simulink model "snac_openloop_SITL"  (R2024a)
settings: Solver=ode1  StartTime=0.0  StopTime=50  FixedStep=0.004  RelTol=1e-3  EnableMultiTasking=on
values from neighbouring files (symbols this model uses):
  x = bsxfun(@plus,x,settings.xoffset)    [NN7.m]
  y = bsxfun(@plus,y,settings.ymin)    [NN7.m]    (also in untitled2.m = r_smooth.r_smooth_1(1:3,:))
undefined symbols (not defined in the file or in its folder): DiscIntNeverNeededParam, vx, vy, vz, yaw, z
libraries: px4uORBlib x6, simulink x3, sharedtransform x1, px4lib x1
settings Model: ExtModeTrigDuration=10  Creator=re606359  LastModifiedBy=re606359
settings SolverCC: PositivePriorityOrder=on
settings OptimizationCC: EnhancedBackFolding=on  PassReuseOutputArgsAs=Individual arguments  ZeroExternalMemoryAtStartup=off  ZeroInternalMemoryAtStartup=off  MaxStackSize=64  OptimizeBlockOrder=speed  DifferentSizesBufferReuse=on  OptimizationCustomize=off  EfficientTunableParamExpr=on
settings DebuggingCC: ParameterTunabilityLossMsg=error
settings HardwareCC: ProdBitPerPointer=32  ProdBitPerSizeT=32  ProdBitPerPtrDiffT=32  ProdLargestAtomicInteger=Long  ProdLargestAtomicFloat=Double  ProdWordSize=32  ProdLongLongMode=on  ProdHWDeviceType=ARM Compatible->ARM Cortex
settings SFSimCC: MATLABDynamicMemAlloc=off  SimTargetLang=C++
settings RTWCC: Description=Embedded Coder  SystemTargetFile=ert.tlc  HardwareBoard=PX4 Host Target  TLCOptions="-aInlineSetEventsForThisBaseRateFcn=TLC_FALSE -aSuppressMultiTaskScheduler=TLC_FALSE  -aRateBasedStepFcn=0"  TemplateMakefile=ert_default_tmf  Toolchain=GNU Tools for PX4 Autopilots  PortableWordSizes=on  TargetLang=C++  GPUComputeCapability=3.5
settings CodeAppCC: ForceParamTrailComments=on  IgnoreCustomStorageClasses=off  OperatorAnnotations=on  SimulinkDataObjDesc=on  SFDataObjDesc=on  InsertBlockDesc=on
settings ERTTargetCC: SupportContinuousTime=on  ExtModeTransport=2  ExtModeStaticAlloc=on  ExtModeMexFile=ext_xcp  ExtModeIntrfLevel=Level2 - Open

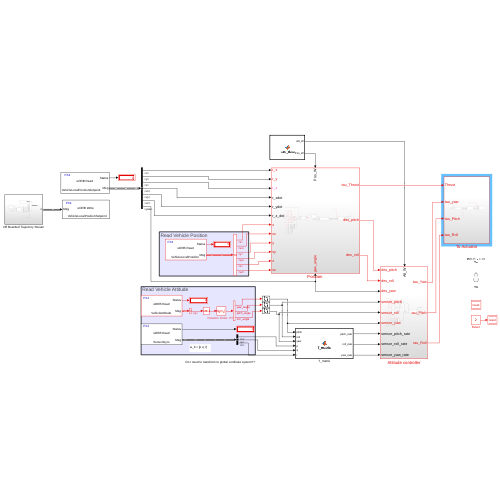
[thumbnail: Simulink's stored preview of the top-level diagram]
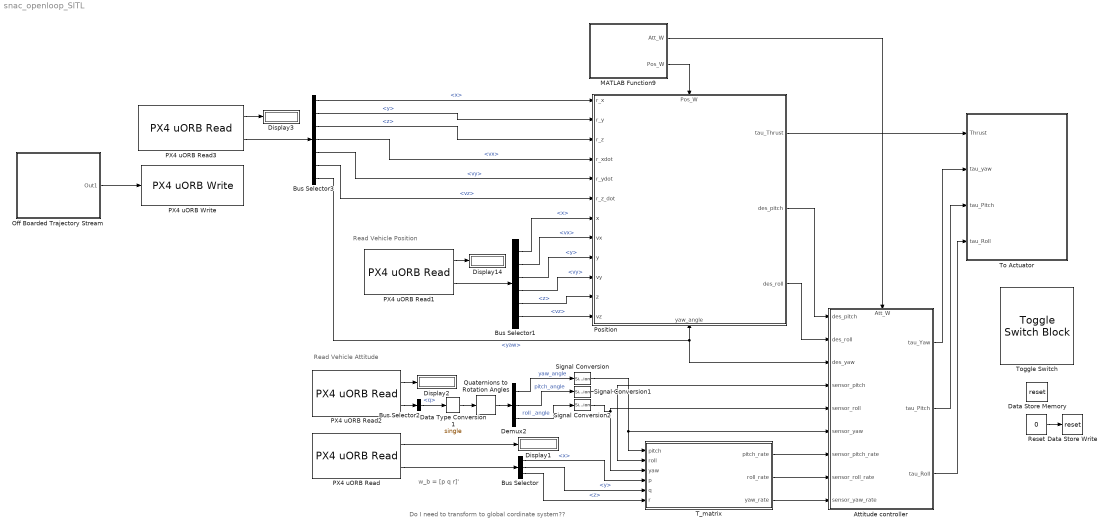
== system snac_openloop_SITL ==
  note: w_b = [p q r]'
  note: Read Vehicle Position
  note: Read Vehicle Attitude
  note: Do I need to transform to global cordinate system??
  Attitude controller : Subsystem
      settings: PortSchema="{\"entries\":[{\"content\":{\"sides\":[{\"content\":{\"connectorIds\":[\"In1\",\"In2\",\"In3\",\"In4\",\"In5\",\"In6\",\"In7\",\"In8\",\"In9\"]},\"type\":\"ConnectorPlacement.EquallySpacedRectSide\",\"uuid\":\"fae962e8-eaa0-4300-aebb-2542e8dc0b9d\"},{\"content\":{\"connectorIds\":[\"Out1\",\"Out2\",\"Out3\"],\"side\":\"RIGHT\"},\"type\":\"ConnectorPlacement.EquallySpacedRectSide\",\"uuid\":\"2ab64516-4178-4987-b105-e2b60ebc653b\"},{\"content\":{\"connectorIds\":[\"In10\"],\"side\":\"TOP\"},\"type\":\"ConnectorPlacement.EquallySpacedRectSide\",\"uuid\":\"8c218eee-bea7-4b7a-ab96-9bd58138bc2f\"},{\"content\":{\"side\":\"BOTTOM\"},\"type\":\"ConnectorPlacement.EquallySpacedRectSide\",\"uuid\":\"12c5faa8-5812-413f-bdcf-aa5ffbd59e54\"}]},\"type\":\"ConnectorPlacement.EquallySpacedConnector\",\"uuid\":\"49b20a1e-3c6c-4df6-a9b5-cb8878061c64\"}],\"packageUris\":[\"http://schema.mathworks.com/mf0/Connector/R2020b\"],\"version\":\"1.0\"}"
  Bus Selector : BusSelector  OutputSignals=x,y,z
  Bus Selector1 : BusSelector  OutputSignals=x,vx,y,vy,z,vz
  Bus Selector2 : BusSelector  OutputSignals=q
  Bus Selector3 : BusSelector  OutputSignals=x,y,z,vx,vy,vz,yaw
  Data Store Write : DataStoreWrite  DataStoreName=reset  IndexOptions=Index vector (dialog)  Indices=1  OutputSizes=1
  Data Store Memory : DataStoreMemory  DataStoreName=reset  ReadBeforeWriteMsg=warning  WriteAfterWriteMsg=warning  WriteAfterReadMsg=warning  ShowAdditionalParam=off  OutDataTypeStr=boolean
  Data Type Conversion1 : DataTypeConversion  OutDataTypeStr=single  SaturateOnIntegerOverflow=off  RndMeth=Floor
  Demux2 : Demux  Outputs=3
  Display{1..3,14} (4 alike) : Display
  MATLAB Function9 : MATLAB Function  TreatAsAtomicUnit=on
  Off Boarded Trajectory Stream : Subsystem
  PX4 uORB Read : px4uORBlib/PX4 uORB Read  uORBTopic=SensorGyro  selectInstance=SensorGyro  SampleTime=-1  BlockingMode=off  BlockTimeout=1e-3
  PX4 uORB Read1 : px4uORBlib/PX4 uORB Read  uORBTopic=VehicleLocalPosition  selectInstance=vehicle_local_position  SampleTime=-1  BlockingMode=off  BlockTimeout=1e-3
  PX4 uORB Read2 : px4uORBlib/PX4 uORB Read  uORBTopic=VehicleAttitude  selectInstance=vehicle_attitude  SampleTime=-1  BlockingMode=off  BlockTimeout=1e-3
  PX4 uORB Read3 : px4uORBlib/PX4 uORB Read  uORBTopic=VehicleLocalPositionSetpoint  selectInstance=VehicleLocalPositionSetpoint  SampleTime=-1  BlockingMode=off  BlockTimeout=1e-3
  PX4 uORB Write : px4uORBlib/PX4 uORB Write  uORBTopic=VehicleLocalPositionSetpoint  selectInstance=VehicleLocalPositionSetpoint  MessageQueueLen=1
  "Position " : Subsystem
      settings: PortSchema="{\"entries\":[{\"content\":{\"sides\":[{\"content\":{\"connectorIds\":[\"In1\",\"In2\",\"In3\",\"In4\",\"In5\",\"In6\",\"In7\",\"In8\",\"In9\",\"In10\",\"In11\",\"In12\"]},\"type\":\"ConnectorPlacement.EquallySpacedRectSide\",\"uuid\":\"96eb1e1d-33f8-43b2-aca1-3a2ea17c97d3\"},{\"content\":{\"connectorIds\":[\"Out1\",\"Out2\",\"Out3\"],\"side\":\"RIGHT\"},\"type\":\"ConnectorPlacement.EquallySpacedRectSide\",\"uuid\":\"68c63f59-0b7f-4dee-beff-edcde1fd911b\"},{\"content\":{\"connectorIds\":[\"In13\"],\"side\":\"TOP\"},\"type\":\"ConnectorPlacement.EquallySpacedRectSide\",\"uuid\":\"695c40b8-e625-4f49-aae8-ed972e1604cc\"},{\"content\":{\"connectorIds\":[\"In14\"],\"side\":\"BOTTOM\"},\"type\":\"ConnectorPlacement.EquallySpacedRectSide\",\"uuid\":\"eed3d45c-6018-4bc3-85c5-6c8aa0ab95cc\"}]},\"type\":\"ConnectorPlacement.EquallySpacedConnector\",\"uuid\":\"b4b28bb8-7674-4138-b24e-55baa1b4cc5c\"}],\"packageUris\":[\"http://schema.mathworks.com/mf0/Connector/R2020b\"],\"version\":\"1.0\"}"
  Quaternions to Rotation Angles : sharedtransform/Quaternions to Rotation Angles  rotationOrder=ZYX  aMode=aMode
  Reset : Constant  Value=0  OutDataTypeStr=boolean  SampleTime=-1
      settings: OpenFcn=|
      | if strcmp('0',get_param(gcb, 'Value'))                        set_param(gcb, 'Value', '1');
      | else
      |             set_param(gcb, 'Value', '0');
      | end
  Signal Conversion : SignalConversion  OverrideOpt=off
  Signal Conversion1 : SignalConversion  OverrideOpt=off
  Signal Conversion2 : SignalConversion  OverrideOpt=off
  T_matrix : MATLAB Function  TreatAsAtomicUnit=on
  To Actuator : Subsystem
  Toggle Switch : ToggleSwitchBlock
      settings: Values={{'Off', 'On'}, [0 1]}
  wires:
  Bus Selector1/3 -> "Position "/9(y)  "<y>"
  Demux2/3 -> Signal Conversion2/1  "roll _angle"
  Quaternions to Rotation Angles/1 -> Demux2/1
  PX4 uORB Read1/1 -> Display14/1
  Bus Selector3/6 -> "Position "/6(r_z_dot)  "<vz>"
  Bus Selector/3 -> T_matrix/6(r)  "<z>"
  Bus Selector1/6 -> "Position "/12(vz)  "<vz>"
  Bus Selector3/4 -> "Position "/4(r_xdot)  "<vx>"
  T_matrix/2(roll_rate) -> Attitude controller/8(sensor_roll_rate)
  T_matrix/1(pitch_rate) -> Attitude controller/7(sensor_pitch_rate)
  Demux2/2 -> Signal Conversion1/1  "pitch_angle"
  "Position "/3(des_roll) -> Attitude controller/2(des_roll)
  Bus Selector1/4 -> "Position "/10(vy)  "<vy>"
  Attitude controller/1(tau_Yaw) -> To Actuator/2(tau_yaw)
  Bus Selector3/2 -> "Position "/2(r_y)  "<y>"
  Bus Selector3/5 -> "Position "/5(r_ydot)  "<vy>"
  PX4 uORB Read2/1 -> Display2/1
  "Position "/1(tau_Thrust) -> To Actuator/1(Thrust)
  PX4 uORB Read2/2 -> Bus Selector2/1
  Bus Selector1/2 -> "Position "/8(vx)  "<vx>"
  PX4 uORB Read1/2 -> Bus Selector1/1
  Bus Selector/1 -> T_matrix/4(p)  "<x>"
  Data Type Conversion1/1 -> Quaternions to Rotation Angles/1
  MATLAB Function9/2(Pos_W) -> "Position "/13(Pos_W)
  PX4 uORB Read3/2 -> Bus Selector3/1
  Signal Conversion1/1 -> Attitude controller/4(sensor_pitch), T_matrix/2(roll)
  Bus Selector/2 -> T_matrix/5(q)  "<y>"
  Bus Selector3/3 -> "Position "/3(r_z)  "<z>"
  "Position "/2(des_pitch) -> Attitude controller/1(des_pitch)
  Bus Selector3/7 -> "Position "/14(yaw_angle), Attitude controller/3(des_yaw)  "<yaw>"
  Demux2/1 -> Signal Conversion/1  "yaw_angle"
  T_matrix/3(yaw_rate) -> Attitude controller/9(sensor_yaw_rate)
  Bus Selector1/1 -> "Position "/7(x)  "<x>"
  PX4 uORB Read/2 -> Bus Selector/1
  Attitude controller/2(tau_Pitch) -> To Actuator/3(tau_Pitch)
  Bus Selector3/1 -> "Position "/1(r_x)  "<x>"
  Reset/1 -> Data Store Write/1
  Bus Selector1/5 -> "Position "/11(z)  "<z>"
  Attitude controller/3(tau_Roll) -> To Actuator/4(tau_Roll)
  PX4 uORB Read/1 -> Display1/1
  Bus Selector2/1 -> Data Type Conversion1/1  "<q>"
  Signal Conversion2/1 -> T_matrix/3(yaw), Attitude controller/5("sensor_roll ")
  PX4 uORB Read3/1 -> Display3/1
  Signal Conversion/1 -> T_matrix/1(pitch), Attitude controller/6(sensor_yaw)
  MATLAB Function9/1(Att_W) -> Attitude controller/10(Att_W)
  Off Boarded Trajectory Stream/1(Out1) -> PX4 uORB Write/1

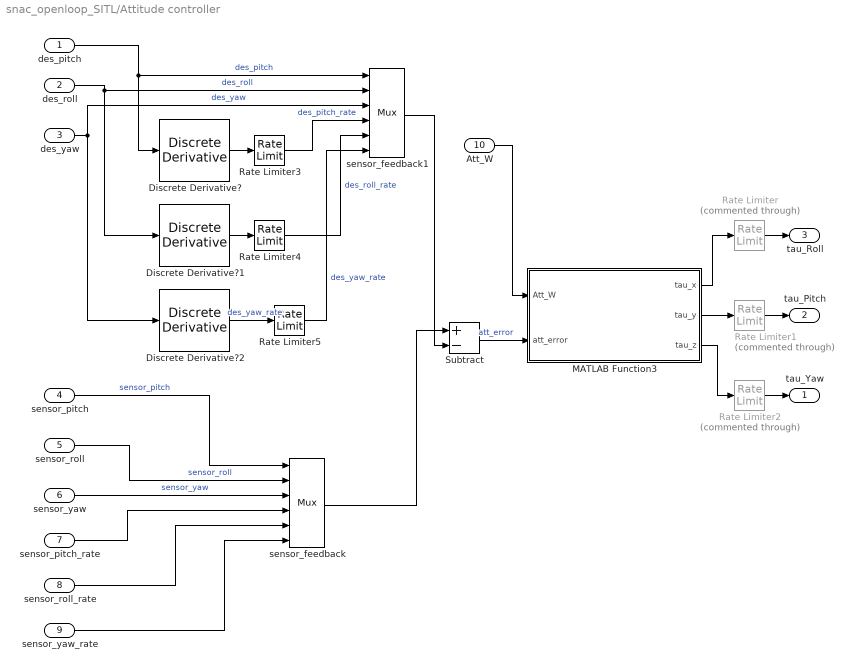
== system snac_openloop_SITL/Attitude controller ==
  des_pitch : Inport  OutDataTypeStr=single
  des_roll : Inport  Port=2  OutDataTypeStr=single
  des_yaw : Inport  Port=3  OutDataTypeStr=single
  sensor_pitch : Inport  Port=4
  "sensor_roll " : Inport  Port=5
  sensor_yaw : Inport  Port=6
  sensor_pitch_rate : Inport  Port=7
  sensor_roll_rate : Inport  Port=8
  sensor_yaw_rate : Inport  Port=9
  Att_W : Inport  Port=10
  Discrete Derivative? : simulink/Discrete/Discrete Derivative  gainval=1.0  ICPrevScaledInput=0.0  OutMin=[-5]  OutMax=[5]  OutDataTypeStr=single  OutputDataTypeScalingMode=single  OutDataType=fixdt(1, 16)  OutScaling=2^-10  DoSatur=off
  Discrete Derivative?1 : simulink/Discrete/Discrete Derivative  gainval=1.0  ICPrevScaledInput=0.0  OutMin=[-5]  OutMax=[5]  OutDataTypeStr=single  OutputDataTypeScalingMode=single  OutDataType=fixdt(1, 16)  OutScaling=2^-10  DoSatur=off
  Discrete Derivative?2 : simulink/Discrete/Discrete Derivative  gainval=1.0  ICPrevScaledInput=0.0  OutMin=[-2]  OutMax=[2]  OutDataTypeStr=single  OutputDataTypeScalingMode=single  OutDataType=fixdt(1, 16)  OutScaling=2^-10  DoSatur=off
  MATLAB Function3 : MATLAB Function  TreatAsAtomicUnit=on
  Rate Limiter : RateLimiter  Commented=through  RisingSlewLimit=2  FallingSlewLimit=-2  SampleTimeMode=inherited
  Rate Limiter1 : RateLimiter  Commented=through  RisingSlewLimit=2  FallingSlewLimit=-2  SampleTimeMode=inherited
  Rate Limiter2 : RateLimiter  Commented=through  RisingSlewLimit=2  FallingSlewLimit=-2  SampleTimeMode=inherited
  Rate Limiter3 : RateLimiter  RisingSlewLimit=2  FallingSlewLimit=-2  SampleTimeMode=inherited
  Rate Limiter4 : RateLimiter  RisingSlewLimit=2  FallingSlewLimit=-2  SampleTimeMode=inherited
  Rate Limiter5 : RateLimiter  RisingSlewLimit=2  FallingSlewLimit=-2  SampleTimeMode=inherited
  Subtract : Sum  Inputs=+-
  sensor_feedback : Mux  Inputs=6
  sensor_feedback1 : Mux  Inputs=6
  tau_Yaw : Outport
  tau_Pitch : Outport  Port=2
  tau_Roll : Outport  Port=3
  wires:
  sensor_pitch/1 -> sensor_feedback/1  "sensor_pitch"
  "sensor_roll "/1 -> sensor_feedback/2  "sensor_roll"
  sensor_yaw/1 -> sensor_feedback/3  "sensor_yaw"
  sensor_pitch_rate/1 -> sensor_feedback/4
  sensor_roll_rate/1 -> sensor_feedback/5
  sensor_yaw_rate/1 -> sensor_feedback/6
  Att_W/1 -> MATLAB Function3/1(Att_W)
  Subtract/1 -> MATLAB Function3/2(att_error)  "att_error"
  des_pitch/1 -> Discrete Derivative?/1, sensor_feedback1/1  "des_pitch"
  des_roll/1 -> Discrete Derivative?1/1, sensor_feedback1/2  "des_roll"
  des_yaw/1 -> Discrete Derivative?2/1, sensor_feedback1/3  "des_yaw"
  Rate Limiter5/1 -> sensor_feedback1/6  "des_yaw_rate"
  Rate Limiter4/1 -> sensor_feedback1/5  "des_roll_rate"
  Rate Limiter3/1 -> sensor_feedback1/4  "des_pitch_rate"
  sensor_feedback/1 -> Subtract/1
  sensor_feedback1/1 -> Subtract/2
  Discrete Derivative?1/1 -> Rate Limiter4/1
  Discrete Derivative?/1 -> Rate Limiter3/1
  Discrete Derivative?2/1 -> Rate Limiter5/1  "des_yaw_rate"
  MATLAB Function3/1(tau_x) -> Rate Limiter/1
  MATLAB Function3/2(tau_y) -> Rate Limiter1/1
  MATLAB Function3/3(tau_z) -> Rate Limiter2/1
  Rate Limiter/1 -> tau_Roll/1
  Rate Limiter1/1 -> tau_Pitch/1
  Rate Limiter2/1 -> tau_Yaw/1

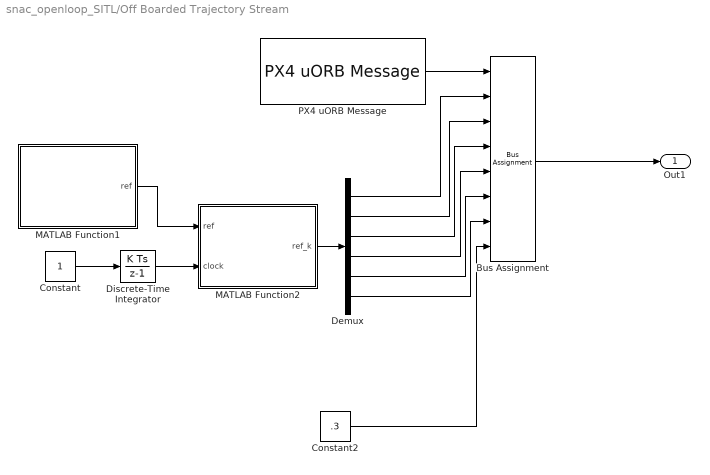
== system snac_openloop_SITL/Off Boarded Trajectory Stream ==
  Bus Assignment : BusAssignment  AssignedSignals=x,y,z,vx,vy,vz,yaw
  Constant : Constant  OutDataTypeStr=single
  Constant2 : Constant  Value=.3  OutDataTypeStr=single
  Demux : Demux  Outputs=6
  Discrete-Time Integrator : DiscreteIntegrator  SampleTime=-1  ICPrevOutput=DiscIntNeverNeededParam  ICPrevScaledInput=DiscIntNeverNeededParam
  MATLAB Function1 : MATLAB Function  TreatAsAtomicUnit=on
  MATLAB Function2 : MATLAB Function  TreatAsAtomicUnit=on
  PX4 uORB Message : px4uORBlib/PX4 uORB Message  uORBTopic=VehicleLocalPositionSetpoint  SampleTime=-1  selectInstance=VehicleLocalPositionSetpoint
  Out1 : Outport
  wires:
  MATLAB Function1/1(ref) -> MATLAB Function2/1(ref)
  Discrete-Time Integrator/1 -> MATLAB Function2/2(clock)
  Demux/2 -> Bus Assignment/3
  Demux/3 -> Bus Assignment/4
  PX4 uORB Message/1 -> Bus Assignment/1
  Demux/1 -> Bus Assignment/2
  Constant/1 -> Discrete-Time Integrator/1
  Demux/4 -> Bus Assignment/5
  Constant2/1 -> Bus Assignment/8
  Demux/5 -> Bus Assignment/6
  Demux/6 -> Bus Assignment/7
  MATLAB Function2/1(ref_k) -> Demux/1
  Bus Assignment/1 -> Out1/1

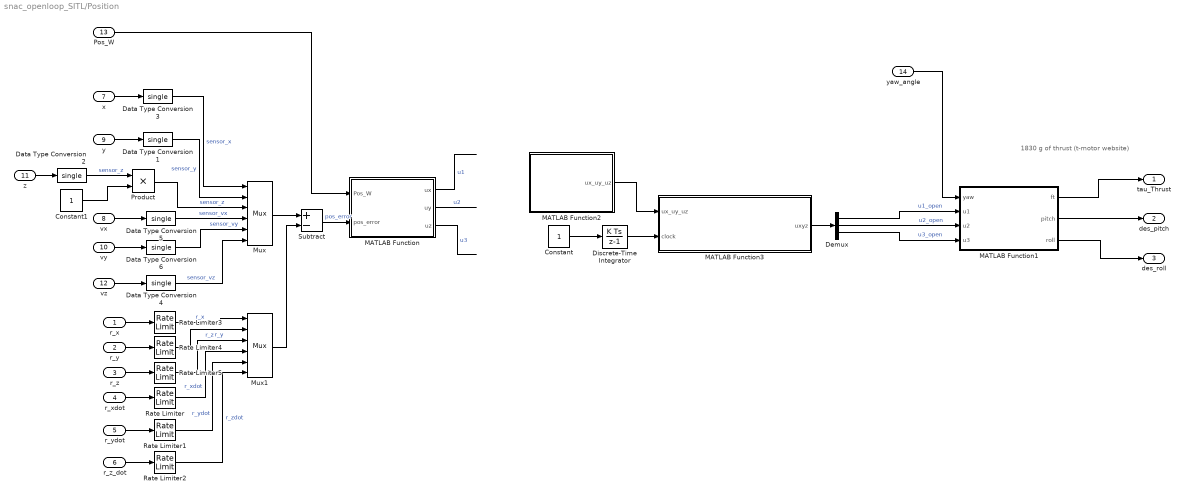
== system snac_openloop_SITL/Position  ==
  note: 1830 g of thrust (t-motor website)
  r_x : Inport
  r_y : Inport  Port=2
  r_z : Inport  Port=3
  r_xdot : Inport  Port=4
  r_ydot : Inport  Port=5
  r_z_dot : Inport  Port=6
  x : Inport  Port=7
  vx : Inport  Port=8
  y : Inport  Port=9
  vy : Inport  Port=10
  z : Inport  Port=11
  vz : Inport  Port=12
  Pos_W : Inport  Port=13
  yaw_angle : Inport  Port=14
  Constant : Constant  OutDataTypeStr=single
  Constant1 : Constant  OutDataTypeStr=single
  Data Type Conversion{1..6} (6 alike) : DataTypeConversion  OutDataTypeStr=single  SaturateOnIntegerOverflow=off  RndMeth=Floor
  Demux : Demux  Outputs=3
  Discrete-Time Integrator : DiscreteIntegrator  SampleTime=-1  ICPrevOutput=DiscIntNeverNeededParam  ICPrevScaledInput=DiscIntNeverNeededParam
  MATLAB Function : MATLAB Function  TreatAsAtomicUnit=on
  MATLAB Function1 : MATLAB Function  TreatAsAtomicUnit=on
  MATLAB Function2 : MATLAB Function  TreatAsAtomicUnit=on
  MATLAB Function3 : MATLAB Function  TreatAsAtomicUnit=on
  Mux : Mux  Inputs=6
  Mux1 : Mux  Inputs=6
  Product : Product
  Rate Limiter{,1..5} (6 alike) : RateLimiter  RisingSlewLimit=15  FallingSlewLimit=-15  SampleTimeMode=inherited
  Subtract : Sum  Inputs=+-
  tau_Thrust : Outport  OutDataTypeStr=single
  des_pitch : Outport  Port=2
  des_roll : Outport  Port=3
  wires:
  z/1 -> Data Type Conversion2/1
  x/1 -> Data Type Conversion3/1
  y/1 -> Data Type Conversion1/1
  vz/1 -> Data Type Conversion4/1
  vx/1 -> Data Type Conversion5/1
  vy/1 -> Data Type Conversion6/1
  Pos_W/1 -> MATLAB Function/1(Pos_W)
  Data Type Conversion3/1 -> Mux/1  "sensor_x"
  Data Type Conversion1/1 -> Mux/2  "sensor_y"
  Data Type Conversion5/1 -> Mux/4  "sensor_vx"
  Data Type Conversion6/1 -> Mux/5  "sensor_vy"
  Data Type Conversion4/1 -> Mux/6  "sensor_vz"
  Mux/1 -> Subtract/1
  Mux1/1 -> Subtract/2
  Subtract/1 -> MATLAB Function/2(pos_error)  "pos_error"
  Demux/1 -> MATLAB Function1/2(u1)  "u1_open"
  Demux/2 -> MATLAB Function1/3(u2)  "u2_open"
  Demux/3 -> MATLAB Function1/4(u3)  "u3_open"
  yaw_angle/1 -> MATLAB Function1/1(yaw)
  r_ydot/1 -> Rate Limiter1/1
  r_z_dot/1 -> Rate Limiter2/1
  r_xdot/1 -> Rate Limiter/1
  Rate Limiter/1 -> Mux1/4  "r_xdot"
  Rate Limiter1/1 -> Mux1/5  "r_ydot"
  Rate Limiter2/1 -> Mux1/6  "r_zdot"
  Data Type Conversion2/1 -> Product/1  "sensor_z"
  Product/1 -> Mux/3  "sensor_z"
  Constant1/1 -> Product/2
  r_x/1 -> Rate Limiter3/1
  Rate Limiter3/1 -> Mux1/1  "r_x"
  r_y/1 -> Rate Limiter4/1
  Rate Limiter4/1 -> Mux1/2  "r_y"
  r_z/1 -> Rate Limiter5/1
  Rate Limiter5/1 -> Mux1/3  "r_z"
  MATLAB Function1/1(ft) -> tau_Thrust/1
  MATLAB Function1/2(pitch) -> des_pitch/1
  MATLAB Function1/3(roll) -> des_roll/1
  MATLAB Function2/1(ux_uy_uz) -> MATLAB Function3/1(ux_uy_uz)
  Discrete-Time Integrator/1 -> MATLAB Function3/2(clock)
  Constant/1 -> Discrete-Time Integrator/1
  MATLAB Function3/1(uxyz) -> Demux/1
  MATLAB Function/3(uz) -> ?  "u3"
  MATLAB Function/1(ux) -> ?  "u1"
  MATLAB Function/2(uy) -> ?  "u2"

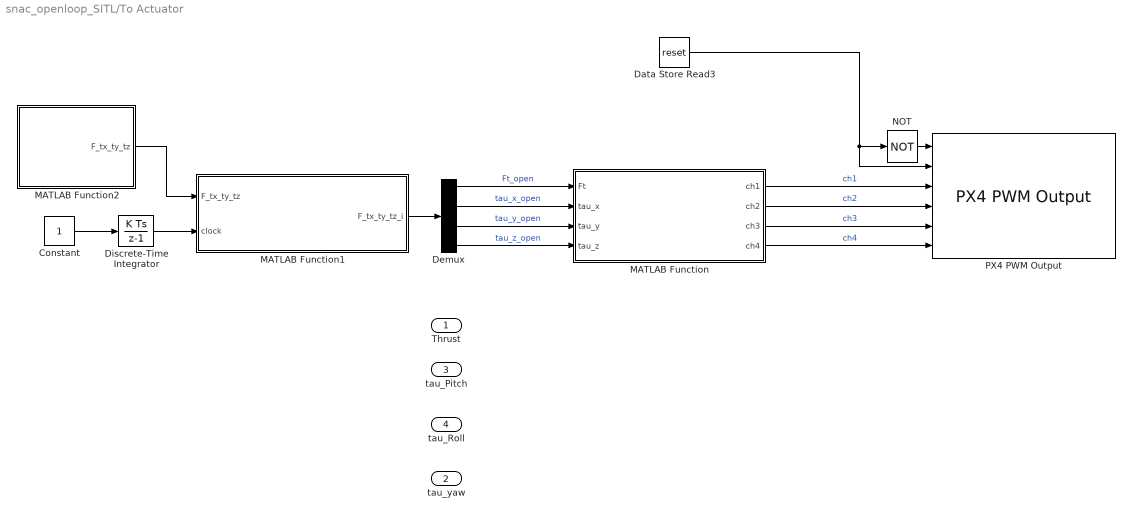
== system snac_openloop_SITL/To Actuator ==
  Thrust : Inport
  tau_yaw : Inport  Port=2
  tau_Pitch : Inport  Port=3
  tau_Roll : Inport  Port=4
  Constant : Constant  OutDataTypeStr=single
  Data Store Read3 : DataStoreRead  DataStoreName=reset  IndexOptions=Index vector (dialog)  Indices=1  OutputSizes=1
  Demux : Demux
  Discrete-Time Integrator : DiscreteIntegrator  SampleTime=-1  ICPrevOutput=DiscIntNeverNeededParam  ICPrevScaledInput=DiscIntNeverNeededParam
  MATLAB Function : MATLAB Function  TreatAsAtomicUnit=on
  MATLAB Function1 : MATLAB Function  TreatAsAtomicUnit=on
  MATLAB Function2 : MATLAB Function  TreatAsAtomicUnit=on
  NOT : Logic  Operator=NOT  IconShape=distinctive  AllPortsSameDT=off  OutDataTypeStr=boolean
  PX4 PWM Output : px4lib/PX4 PWM Output  pwmDevice=Main  pwmChannel1_=on  pwmChannel2_=on  pwmChannel3_=on  pwmChannel4_=on  pwmChannel5_=off  pwmChannel6_=off  pwmChannel7_=off  pwmChannel8_=off
  wires:
  NOT/1 -> PX4 PWM Output/1
  Data Store Read3/1 -> PX4 PWM Output/2, NOT/1
  MATLAB Function/1(ch1) -> PX4 PWM Output/3  "ch1"
  MATLAB Function/2(ch2) -> PX4 PWM Output/4  "ch2"
  MATLAB Function/3(ch3) -> PX4 PWM Output/5  "ch3"
  MATLAB Function/4(ch4) -> PX4 PWM Output/6  "ch4"
  MATLAB Function2/1(F_tx_ty_tz) -> MATLAB Function1/1(F_tx_ty_tz)
  Constant/1 -> Discrete-Time Integrator/1
  Discrete-Time Integrator/1 -> MATLAB Function1/2(clock)
  MATLAB Function1/1(F_tx_ty_tz_i) -> Demux/1
  Demux/1 -> MATLAB Function/1(Ft)  "Ft_open"
  Demux/2 -> MATLAB Function/2(tau_x)  "tau_x_open"
  Demux/3 -> MATLAB Function/3(tau_y)  "tau_y_open"
  Demux/4 -> MATLAB Function/4(tau_z)  "tau_z_open"

== matlab function snac_openloop_SITL/Attitude controller/MATLAB Function3 ==
  data: Att_W input; att_error input; tau_x output; tau_y output; tau_z output
function [tau_x, tau_y, tau_z] = attitude_control(Att_W, att_error)
           
        dt = single(0.004);
        Ix = single(2); Iy = single(2); Iz = single(4);
        Attitude_R = diag([1,1,1]);
        Attitude_G = [0 0 0; 0 0 0; 0 0 0; 1/Ix 0 0; 0 1/Iy 0; 0 0 1/Iz]*dt;


        torques = -Attitude_R^-1 * Attitude_G' * Att_W' * Basis_Func_84(att_error(:));
        tau_x = single(zeros(1,1));
        tau_y = single(zeros(1,1));
        tau_z = single(zeros(1,1));
        tau_x = (torques(1));
        tau_y = (torques(2));
        tau_z = (torques(3));

        max_tau = single(8.6);
        
        % if tau_x > max_tau
        %     tau_x = single(max_tau);
        % elseif tau_x < -max_tau
        %     tau_x = single(-max_tau);
        % end
        % if tau_y > max_tau
        %     tau_y = single(max_tau);
        % elseif tau_y < -max_tau
        %     tau_y = single(-max_tau);
        % end
        % if tau_z > max_tau
        %     tau_z = single(max_tau);
        % elseif tau_z < -max_tau
        %     tau_z = single(-max_tau);
        % end

end

function out = Basis_Func_84(x)
    % assert( isequal(size(x), [6, 1]),'Input must be a 6x1 matrix of real finite doubles.');
x1 = x(1);
x2 = x(2);
x3 = x(3);
x4 = x(4);
x5 = x(5);
x6 = x(6);

out = [ 
    [ones(1,length(x(1,:)))];
    x1
    x2
    x3
    x4
    x5
    x6
    % polynomial terms
    x1^2
    x2^2
    x3^2
    x4^2
    x5^2
    x6^2
    x1^3
    x2^3
    x3^3
    x4^3
    x5^3
    x6^3
    x1^4
    x2^4
    x3^4
    x4^4
    x5^4
    x6^4
    % 2 - term combinations
    x1*x2
    x1*x3
    x1*x4
    x2*x3
    x1*x5
    x2*x4
    x1*x6
    x2*x5
    x3*x4
    x2*x6
    x3*x5
    x3*x6
    x4*x5
    x4*x6
    x5*x6
    % 3 term combinations
    x1*x2*x3
    x1*x2*x4
    x1*x2*x5
    x1*x2*x6
    x1*x3*x4
    x1*x3*x5
    x1*x3*x6
    x1*x4*x5
    x1*x4*x6
    x1*x5*x6
    x2*x3*x4
    x2*x3*x5
    x2*x3*x6
    x2*x4*x5
    x2*x4*x6
    x2*x5*x6
    x3*x4*x5
    x3*x4*x6
    x3*x5*x6
    x4*x5*x6
    % 4 term combinations
    x1*x2*x3*x4
    x1*x2*x3*x5
    x1*x2*x3*x6
    x1*x2*x4*x5
    x1*x2*x4*x6
    x1*x2*x5*x6
    x1*x3*x4*x5
    x1*x3*x4*x6
    x1*x3*x5*x6
    x1*x4*x5*x6
    x2*x3*x4*x5
    x2*x3*x4*x6
    x2*x3*x5*x6
    x2*x4*x5*x6
    x3*x4*x5*x6
    % 5 and 6 term combinations
    x1*x2*x3*x4*x5
    x1*x2*x3*x4*x6
    x1*x2*x3*x5*x6
    x1*x2*x4*x5*x6
    x1*x3*x4*x5*x6
    x2*x3*x4*x5*x6
    x1*x2*x3*x4*x5*x6
    % 2 terms with 1 squared
    x1*x2^2
    x1^2*x2
    x1*x3^2
    x1^2*x3
    x1*x4^2
    x1^2*x4
    x1*x5^2
    x1^2*x5
    x1*x6^2
    x1^2*x6
    x2*x3^2
    x2^2*x3
    x2*x4^2
    x2^2*x4
    x2*x5^2
    x2^2*x5
    x2*x6^2
    x2^2*x6
    x3*x4^2
    x3^2*x4
    x3*x5^2
    x3^2*x5
    x3*x6^2
    x3^2*x6
    x4*x5^2
    x4^2*x5
    x4*x6^2
    x4^2*x6
    x5*x6^2
    x5^2*x6
    % 3 terms with 1 squared
    x1*x2*x3^2
    x1*x2^2*x3
    x1^2*x2*x3
    x1*x2*x4^2
    x1*x2^2*x4
    x1^2*x2*x4
    x1*x2*x5^2
    x1*x2^2*x5
    x1^2*x2*x5
    x1*x2*x6^2
    x1*x2^2*x6
    x1^2*x2*x6
    x1*x3*x4^2
    x1*x3^2*x4
    x1^2*x3*x4
    x1*x3*x5^2
    x1*x3^2*x5
    x1^2*x3*x5
    x1*x3*x6^2
    x1*x3^2*x6
    x1^2*x3*x6
    x1*x4*x5^2
    x1*x4^2*x5
    x1^2*x4*x5
    x1*x4*x6^2
    x1*x4^2*x6
    x1^2*x4*x6
    x1*x5*x6^2
    x1*x5^2*x6
    x1^2*x5*x6
    x2*x3*x4^2
    x2*x3^2*x4
    x2^2*x3*x4
    x2*x3*x5^2
    x2*x3^2*x5
    x2^2*x3*x5
    x2*x3*x6^2
    x2*x3^2*x6
    x2^2*x3*x6
    x2*x4*x5^2
    x2*x4^2*x5
    x2^2*x4*x5
    x2*x4*x6^2
    x2*x4^2*x6
    x2^2*x4*x6
    x2*x5*x6^2
    x2*x5^2*x6
    x2^2*x5*x6
    x3*x4*x5^2
    x3*x4^2*x5
    x3^2*x4*x5
    x3*x4*x6^2
    x3*x4^2*x6
    x3^2*x4*x6
    x3*x5*x6^2
    x3*x5^2*x6
    x3^2*x5*x6
    x4*x5*x6^2
    x4*x5^2*x6
    x4^2*x5*x6
    % % 2 terms with both squared
    % x1^2*x2^2
    % x1^2*x3^2
    % x1^2*x4^2
    % x2^2*x3^2
    % x1^2*x5^2
    % x2^2*x4^2
    % x1^2*x6^2
    % x2^2*x5^2
    % x3^2*x4^2
    % x2^2*x6^2
    % x3^2*x5^2
    % x3^2*x6^2
    % x4^2*x5^2
    % x4^2*x6^2
    % x5^2*x6^2
    % % 3 terms with all squared
    % (x1*x2*x3)^2
    % (x1*x2*x4)^2
    % (x1*x2*x5)^2
    % (x1*x2*x6)^2
    % (x1*x3*x4)^2
    % (x1*x3*x5)^2
    % (x1*x3*x6)^2
    % (x1*x4*x5)^2
    % (x1*x4*x6)^2
    % (x1*x5*x6)^2
    % (x2*x3*x4)^2
    % (x2*x3*x5)^2
    % (x2*x3*x6)^2
    % (x2*x4*x5)^2
    % (x2*x4*x6)^2
    % (x2*x5*x6)^2
    % (x3*x4*x5)^2
    % (x3*x4*x6)^2
    % (x3*x5*x6)^2
    % (x4*x5*x6)^2
 ];
end

== matlab function snac_openloop_SITL/T_matrix ==
  data: pitch input; pitch_rate output; roll input; yaw input; p input; q input; r input; roll_rate output; yaw_rate output
function [pitch_rate, roll_rate, yaw_rate] = T_matrix(pitch, roll, yaw, p, q, r)

    w = [1,     sin(pitch)*tan(roll),       cos(pitch)*tan(roll)
        0,      cos(pitch),                 -sin(pitch)
        0,      sin(pitch)/cos(roll),       cos(pitch)/cos(roll)]*[p; q; r];
    pitch_rate= w(1);
    roll_rate= w(2);
    yaw_rate= w(3);

end

== matlab function snac_openloop_SITL/Off Boarded Trajectory Stream/MATLAB Function1 ==
  data: ref output
function ref = load_ref()

    data = coder.load('reference_SITL.mat', 'ref_states');    
    % Extract and convert the matrices to double
    ref = single(data.ref_states);


              

end

== matlab function snac_openloop_SITL/Off Boarded Trajectory Stream/MATLAB Function2 ==
  data: ref_k output; ref input; clock input
function ref_k = stream_ref(ref, clock)
    sample_time = 0.004;
    index = round(clock / sample_time) + 1; % Convert time to index
    index = min(index, size(ref, 2)); % Prevent index overflow
    ref_k = ref(:, index);
    % ref_k(3) = -1*ref(3);

end

== matlab function snac_openloop_SITL/To Actuator/MATLAB Function ==
  data: Ft input; ch1 output; tau_x input; tau_y input; tau_z input; ch2 output; ch3 output; ch4 output
function [ch1, ch2, ch3, ch4] = actuator_mapping(Ft, tau_x, tau_y, tau_z)

% LARGE DRONE
    % assume Min thrust the motor can reliably genorate is 5N
    % max thrust of T-motor:MN 4010 KV370 with 14x4.8 prop is 17.85 N
    % PWM_i = 1000 + (((Ti - Tmin) / Tmax-Tmin) * 1000 )
    r = single(.24);
    b = single(0.01); % (drag coef)
    T_min = single(2);
    T_max = single(18);
    Tmin = uint16(2);
    Tmax = uint16(18);
    MAX_PWM = uint16(2000);
    MIN_PWM = uint16(1000);

 % Small drone
    % assume Min thrust the motor can reliably genorate is .1N
    % max thrust of 4N
    % PWM_i = 1000 + (((Ti - Tmin) / Tmax-Tmin) * 1000 )
    % r = .15;
    % b = 0.01; % (drag coef)
    T1 = (Ft - tau_x/(2*r) - tau_y/(2*r) + tau_z/(4*b)) / 4;
    T2 = (Ft - tau_x/(2*r) + tau_y/(2*r) + tau_z/(4*b)) / 4;
    T3 = (Ft + tau_x/(2*r) - tau_y/(2*r) - tau_z/(4*b)) / 4;
    T4 = (Ft + tau_x/(2*r) + tau_y/(2*r) - tau_z/(4*b)) / 4;

    if T1 > T_max
        T1 = T_max;
    elseif T1 < T_min
        T1 = T_min;
    end
    if T2 > T_max
        T2 = T_max;
    elseif T2 < T_min
        T2 = T_min;
    end
    if T3 > T_max
        T3 = T_max;
    elseif T3 < T_min
        T3 = T_min;
    end
    if T4 > T_max
        T4 = T_max;
    elseif T4 < T_min
        T4 = T_min;
    end

    T1 = uint16(round(T1));
    T2 = uint16(round(T2));
    T3 = uint16(round(T3));
    T4 = uint16(round(T4));

    ch1 = 1000 + (((T1 - Tmin ) / (Tmax-Tmin)) * 1000  );
    ch2 = 1000 + (((T2 - Tmin) / (Tmax-Tmin)) * 1000  );
    ch3 = 1000 + (((T3 - Tmin) / (Tmax-Tmin)) * 1000  );
    ch4 = 1000 + (((T4 - Tmin) / (Tmax-Tmin)) * 1000 );



    if ch1 > MAX_PWM
        ch1 = MAX_PWM;
    elseif ch1 < MIN_PWM
        ch1 = MIN_PWM;
    end
    if ch2 > MAX_PWM
        ch2 = MAX_PWM;
    elseif ch2 < MIN_PWM
        ch2 = MIN_PWM;
    end
    if ch3 > MAX_PWM
        ch3 = MAX_PWM;
    elseif ch3 < MIN_PWM
        ch3 = MIN_PWM;
    end
    if ch4 > MAX_PWM
        ch4 = MAX_PWM;
    elseif ch4 < MIN_PWM
        ch4 = MIN_PWM;
    end


end

== matlab function snac_openloop_SITL/Position /MATLAB Function2 ==
  data: ux_uy_uz output
function ux_uy_uz = load_uxyz()

    data = coder.load('open_loop_controls.mat', 'u1_u2_u3');    
    % Extract and convert the matrices to double
    ux_uy_uz = single(data.u1_u2_u3);

              

end

== matlab function snac_openloop_SITL/Position /MATLAB Function3 ==
  data: uxyz output; ux_uy_uz input; clock input
function uxyz = stream_position_controls(ux_uy_uz, clock)
    sample_time = 0.004;
    index = round(clock / sample_time) + 1; % Convert time to index
    index = min(index, size(ux_uy_uz, 2)); % Prevent index overflow
    uxyz = ux_uy_uz(:, index);

end

== matlab function snac_openloop_SITL/To Actuator/MATLAB Function1 ==
  data: F_tx_ty_tz_i output; F_tx_ty_tz input; clock input
function F_tx_ty_tz_i = stream_controls(F_tx_ty_tz, clock)
    sample_time = 0.004;
    index = round(clock / sample_time) + 1; % Convert time to index
    index = min(index, size(F_tx_ty_tz, 2)); % Prevent index overflow
    F_tx_ty_tz_i = F_tx_ty_tz(:, index);

end

== matlab function snac_openloop_SITL/To Actuator/MATLAB Function2 ==
  data: F_tx_ty_tz output
function F_tx_ty_tz = load_F_tx_ty_tz()

    data = coder.load('open_loop_controls.mat', 'F_tx_ty_tz');    
    % Extract and convert the matrices to double
    F_tx_ty_tz = single(data.F_tx_ty_tz);

              

end

== matlab function snac_openloop_SITL/Position /MATLAB Function ==
  data: Pos_W input; pos_error input; ux output; uy output; uz output
function [ux, uy, uz] = position_control(Pos_W, pos_error)
        
        dt = single(0.004);
        Position_R = single(diag([10000,10000,10000]) );
        Position_G = @(x) [0 0 0; 0 0 0; 0 0 0; -1 0 0; 0 -1 0; 0 0 -1] * dt;

        uxyz = -Position_R^-1 * Position_G( pos_error )' * Pos_W' * Basis_Func_pos(pos_error );
        
        ux = single(zeros(1,1));
        uy = single(zeros(1,1));
        uz = single(zeros(1,1));
        
        ux = (uxyz(1));
        uy = (uxyz(2));
        uz = (uxyz(3));
        


end

function out = Basis_Func_pos(x)
    % assert( isequal(size(x), [6, 1]),'Input must be a 6x1 matrix of real finite doubles.');
x1 = x(1);
x2 = x(2);
x3 = x(3);
x4 = x(4);
x5 = x(5);
x6 = x(6);

out = [1
    x1
    x2
    x3
    x4
    x5
    x6
    x1^2
    x2^2
    x3^2
    x4^2
    x5^2
    x6^2
 ];
end

== matlab function snac_openloop_SITL/Position /MATLAB Function1 ==
  data: yaw input; u1 input; u2 input; ft output; u3 input; pitch output; roll output
function [ft, pitch, roll] = borna_sys_solve(yaw, u1, u2, u3)

% make this more mem efficient later
    ft_max = single(72);
    m = single(3.2);
    ft = single(zeros(1,1));
    pitch = single(zeros(1,1));
    pitch_max = single(pi/6);
    roll = single(zeros(1,1));
    roll_max = single(pi/6);

    % if psi <= 0.001 && psi >= -0.001
    %     psi = single(0.001);
    % end
    u1 = -u1;
    u2 = -u2;
    u3 = -u3;
    a = sin(yaw);
    b = cos(yaw);

    A = u1 / (u3);
    B = u2 / (u3);
    C = (a*A - b*B) / ( (a^2) + (b^2)) ;

    roll = single(atan( (B + b*C) / a ));
    pitch = single(atan( C * cos(roll) )); 

    if pitch>pitch_max
        pitch = pitch_max;
    elseif pitch<-pitch_max
        pitch = -pitch_max;
    end

    if roll>roll_max
        roll = roll_max;
    elseif roll<-roll_max
        roll = -roll_max;
    end
    
    ft = ( m / (cos(pitch)*cos(roll)) ) * (-u3);

    % if ft< 0 
    %     ft = single(0);
    % elseif ft> ft_max
    %         ft = ft_max;
    % end


end

== matlab function snac_openloop_SITL/MATLAB Function9 ==
  data: Att_W output; Pos_W output
function [Att_W, Pos_W] = load_data()

    data_thing = coder.load('trained_weights.mat', 'Position_W', 'Attitude_W');    
    % Extract and convert the matrices to double
    Pos_W = single(data_thing.Position_W);
    Att_W = single(data_thing.Attitude_W);
                


end
